simulink model "mpcACCsystem_MPCBlock"  (R2025a)
settings: Solver=VariableStepAuto  StartTime=0.0  StopTime=80  RelTol=1e-3
undefined symbols (not defined in the file or in its folder): t_gap, Ts, v0_ego, v0_lead, v_set, x0_ego, x0_lead
libraries: mpclib x2
settings Model: Creator=amyyang  LastModifiedBy=amyyang

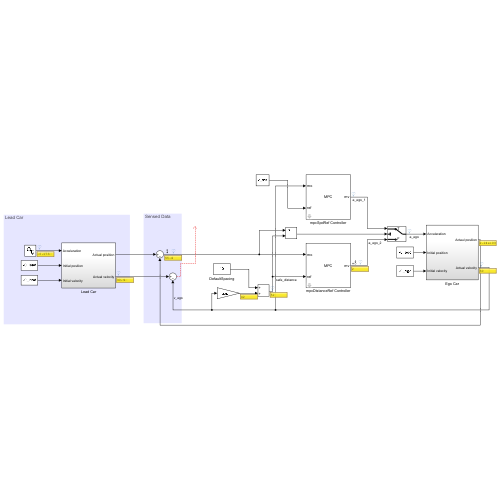
[thumbnail: Simulink's stored preview of the top-level diagram]
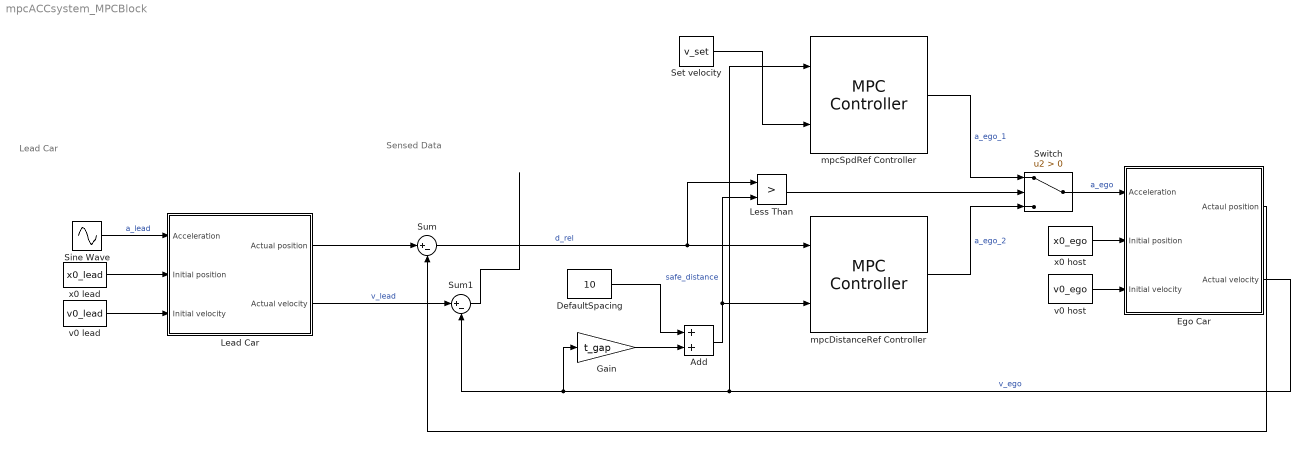
== system mpcACCsystem_MPCBlock ==
  note: Sensed Data
  note: Lead Car
  Add : Sum
  DefaultSpacing : Constant  Value=10  SampleTime=Ts
  Ego Car : Subsystem
  Gain : Gain  Gain=t_gap
  Lead Car : Subsystem
  Less Than : RelationalOperator  Operator=>  OutDataTypeStr=boolean  RndMeth=Simplest  InputSameDT=off
  Set velocity : Constant  Value=v_set  SampleTime=Ts
  Sine Wave : Sin  Amplitude=0.6  Frequency=0.2  SampleTime=Ts
  Sum : Sum  Inputs=|+-
  Sum1 : Sum  Inputs=|+-
  Switch : Switch  Criteria=u2 > Threshold  SaturateOnIntegerOverflow=off  InputSameDT=off
  mpcDistanceRef Controller : mpclib/MPC Controller  SCDEnableBlockLinearizationSpecification=on  mpcobj=mpcDistanceRef  is_multiple=0  enable_value=0  return_u0=off  updateMPCinCallerWorkspace=on  md_inport=off  mv_inport=off  uref_inport=off  return_cost=off  return_mvseq=off  return_qpstatus=off  return_xseq=off  return_state=off  return_ovseq=off  state_inport=off  umin_inport=off  umax_inport=off  ymin_inport=off  ymax_inport=off  cc_inport=off  ywt_inport=off  uwt_inport=off  duwt_inport=off  rhoeps_inport=off  pm_inport=off  MaximumP=10  HorizonChoice=FixedHorizon  n_ts=0.1  n_p=30  n_mv=1  n_md=0  n_ud=0  n_mo=1  n_uo=0  BlockDataType=double  SampleTimeInherited=off  switch_inport=off
  mpcSpdRef Controller : mpclib/MPC Controller  SCDEnableBlockLinearizationSpecification=on  mpcobj=mpcSpdRef  is_multiple=0  enable_value=0  return_u0=off  updateMPCinCallerWorkspace=on  md_inport=off  mv_inport=off  uref_inport=off  return_cost=off  return_mvseq=off  return_qpstatus=off  return_xseq=off  return_state=off  return_ovseq=off  state_inport=off  umin_inport=off  umax_inport=off  ymin_inport=off  ymax_inport=off  cc_inport=off  ywt_inport=off  uwt_inport=off  duwt_inport=off  rhoeps_inport=off  pm_inport=off  MaximumP=10  HorizonChoice=FixedHorizon  n_ts=0.1  n_p=30  n_mv=1  n_md=0  n_ud=0  n_mo=1  n_uo=0  BlockDataType=double  SampleTimeInherited=off  switch_inport=off
  v0 host : Constant  Value=v0_ego  SampleTime=Ts
  v0 lead : Constant  Value=v0_lead  SampleTime=Ts
  x0 host : Constant  Value=x0_ego  SampleTime=Ts
  x0 lead : Constant  Value=x0_lead  SampleTime=Ts
  wires:
  mpcDistanceRef Controller/1 -> Switch/3  "a_ego_2"
  v0 host/1 -> Ego Car/3(Initial velocity)
  x0 host/1 -> Ego Car/2(Initial position)
  Sum/1 -> Less Than/1, mpcDistanceRef Controller/1  "d_rel"
  Lead Car/2(Actual velocity) -> Sum1/1  "v_lead"
  Sine Wave/1 -> Lead Car/1(Acceleration)  "a_lead"
  Sum1/1 -> ?
  Lead Car/1(Actual position) -> Sum/1
  Ego Car/2(Actual velocity) -> mpcSpdRef Controller/1, Gain/1, Sum1/2  "v_ego"
  Ego Car/1(Actaul position) -> Sum/2
  v0 lead/1 -> Lead Car/3(Initial velocity)
  x0 lead/1 -> Lead Car/2(Initial position)
  Set velocity/1 -> mpcSpdRef Controller/2
  DefaultSpacing/1 -> Add/1
  Gain/1 -> Add/2
  Add/1 -> Less Than/2, mpcDistanceRef Controller/2  "safe_distance"
  mpcSpdRef Controller/1 -> Switch/1  "a_ego_1"
  Switch/1 -> Ego Car/1(Acceleration)  "a_ego"
  Less Than/1 -> Switch/2

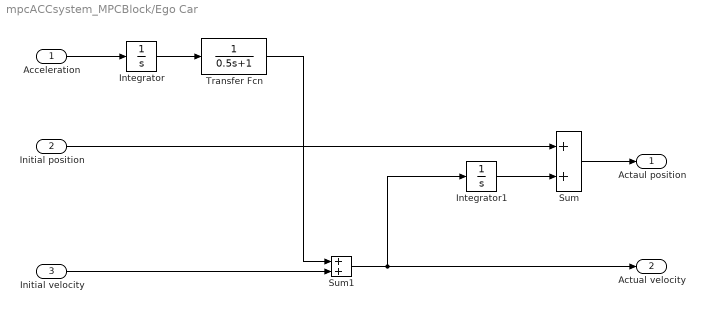
== system mpcACCsystem_MPCBlock/Ego Car ==
  Acceleration : Inport
  Initial position : Inport  Port=2
  Initial velocity : Inport  Port=3
  Integrator : Integrator
  Integrator1 : Integrator
  Sum : Sum
  Sum1 : Sum
  Transfer Fcn : TransferFcn  Denominator=[0.5 1]
  Actaul position : Outport  VectorParamsAs1DForOutWhenUnconnected=off
  Actual velocity : Outport  Port=2  VectorParamsAs1DForOutWhenUnconnected=off
  wires:
  Integrator1/1 -> Sum/2
  Initial position/1 -> Sum/1
  Acceleration/1 -> Integrator/1
  Integrator/1 -> Transfer Fcn/1
  Transfer Fcn/1 -> Sum1/1
  Sum/1 -> Actaul position/1
  Initial velocity/1 -> Sum1/2
  Sum1/1 -> Actual velocity/1, Integrator1/1

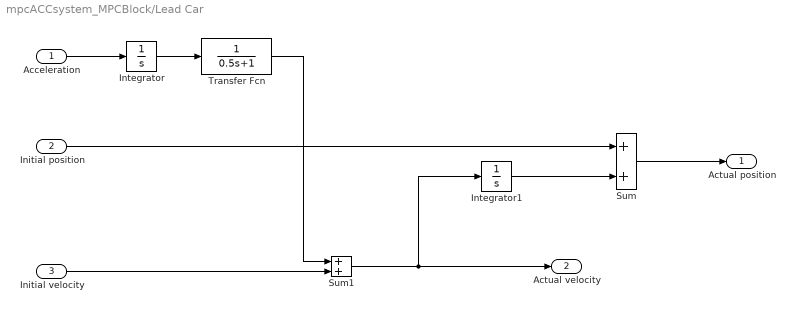
== system mpcACCsystem_MPCBlock/Lead Car ==
  Acceleration : Inport
  Initial position : Inport  Port=2
  Initial velocity : Inport  Port=3
  Integrator : Integrator
  Integrator1 : Integrator
  Sum : Sum
  Sum1 : Sum
  Transfer Fcn : TransferFcn  Denominator=[0.5 1]
  Actual position : Outport  VectorParamsAs1DForOutWhenUnconnected=off
  Actual velocity : Outport  Port=2  VectorParamsAs1DForOutWhenUnconnected=off
  wires:
  Integrator1/1 -> Sum/2
  Initial position/1 -> Sum/1
  Acceleration/1 -> Integrator/1
  Sum1/1 -> Actual velocity/1, Integrator1/1
  Integrator/1 -> Transfer Fcn/1
  Sum/1 -> Actual position/1
  Initial velocity/1 -> Sum1/2
  Transfer Fcn/1 -> Sum1/1
